simulink model "kadai4"  (R2019b)
settings: Solver=VariableStepAuto  StartTime=0.0  StopTime=10.0  RelTol=1e-3
values from neighbouring files (symbols this model uses):
  Kiv = 1    [ex01.m]
  Kpv = 1    [ex01.m]
settings Model: Creator=ryoga  LastModifiedBy=ryoga

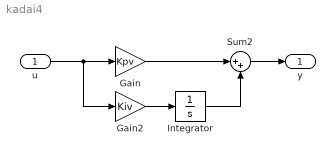
== system kadai4 ==
  u : Inport
  Gain : Gain  Gain=Kpv
  Gain2 : Gain  Gain=Kiv
  Integrator : Integrator
  Sum2 : Sum  Inputs=|++
  y : Outport
  wires:
  Sum2/1 -> y/1
  u/1 -> Gain2/1, Gain/1
  Gain2/1 -> Integrator/1
  Integrator/1 -> Sum2/2
  Gain/1 -> Sum2/1
